simulink model "es_1"  (R2014a)
settings: Solver=ode45  StartTime=0.0  StopTime=10.0  RelTol=1e-3
values from neighbouring files (symbols this model uses):
  A1 = 5.5*10^-3    (= 0.0055)    [es.m]
libraries: cstblocks x4, simulink x1
settings Model: Creator=matdo  LastModifiedBy=matdo

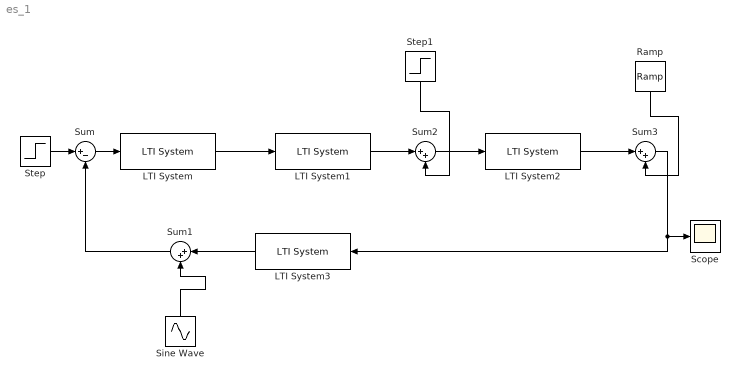
== system es_1 ==
  LTI System : cstblocks/LTI System  sys=C  IC=[]
  LTI System1 : cstblocks/LTI System  sys=A  IC=[]
  LTI System2 : cstblocks/LTI System  sys=Gp  IC=[]
  LTI System3 : cstblocks/LTI System  sys=Kr  IC=[]
  Ramp : simulink/Sources/Ramp  slope=1  start=0  X0=0
  Scope : Scope
  Sine Wave : Sin  SampleTime=0
  Step : Step  SampleTime=0
  Step1 : Step  After=A1  SampleTime=0
  Sum : Sum  Inputs=|+-
  Sum1 : Sum  Inputs=|++
  Sum2 : Sum  Inputs=|++
  Sum3 : Sum  Inputs=|++
  wires:
  LTI System/1 -> LTI System1/1
  Step/1 -> Sum/1
  Sum/1 -> LTI System/1
  Sine Wave/1 -> Sum1/2
  LTI System3/1 -> Sum1/1
  Sum1/1 -> Sum/2
  Step1/1 -> Sum2/2
  Sum2/1 -> LTI System2/1
  LTI System1/1 -> Sum2/1
  Ramp/1 -> Sum3/2
  LTI System2/1 -> Sum3/1
  Sum3/1 -> LTI System3/1, Scope/1
